simulink model "image_processing_system"  (Simulink 7.6)
settings: Solver=FixedStepDiscrete  StartTime=0.0  StopTime=inf  FixedStep=(1/19200)  RelTol=1e-3
undefined symbols (not defined in the file or in its folder): none, serial, videoinput
libraries: instrumentlib x2, vipsnks x1, imaqlib x1, vipstatistics x1
settings Model: Creator=jdoke  LastModifiedBy=Team10
settings DataIOCC: LimitDataPoints=off
settings OptimizationCC: InlineParams=on
settings DebuggingCC: SolverPrmCheckMsg=none  StrictBusMsg=Warning
settings ModelReferenceCC: ModelReferenceNumInstancesAllowed=Single

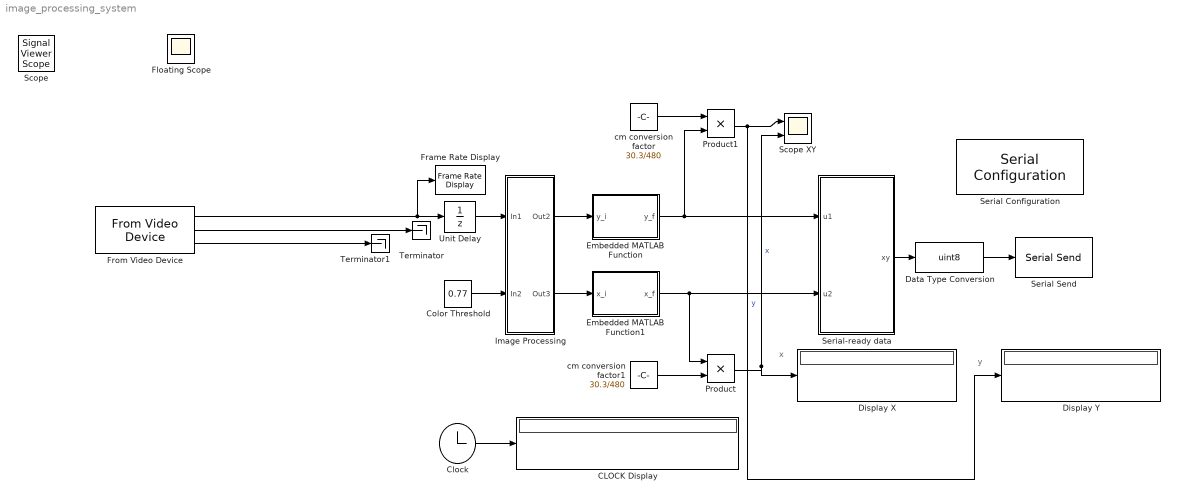
== system image_processing_system ==
  note: y
  note: x
  CLOCK Display : Display
  Clock : Clock
      settings: Decimation=10
  Color Threshold : Constant  Value=0.77
  Data Type Conversion : DataTypeConversion  OutDataTypeStr=uint8
  Display X : Display
  Display Y : Display
  Embedded MATLAB Function : Stateflow chart  TreatAsAtomicUnit=on
  Embedded MATLAB Function1 : Stateflow chart  TreatAsAtomicUnit=on
  Frame Rate Display : vipsnks/Frame Rate Display  DialogController=vipDDGCreate  DialogControllerArgs=DataTag0  UpdateRate=10
  From Video Device : imaqlib/From Video Device  DialogController=imaqcreatedialog  DialogControllerArgs=DataTag2  DeviceMenu=winvideo 1 (PC VGA Camer@ Plus)  Device=winvideo 1 (PC VGA Camer@ Plus)  ObjConstructor=videoinput('winvideo', 1)  VideoFormatMenu=RGB24_640x480  VideoFormat=RGB24_640x480  VideoSource=input1  ROIPosition=[0 0 480 480]  EnableHWTrigger=off  TriggerConfiguration=none/none  SampleTime=1/192  OutputPortsMode=Separate color signals  DataType=single  CanDoHWTrigger=no  ReturnedColorSpace=rgb  BlockHandle=31.001  ROIWidth=480  ROIHeight=480  ROIColumn=0  ROIRow=0  EngXMLPath=C:\Program Files\MATLAB\R2010b\toolbox\imaq\imaq\private  DevXMLPath=C:\Program Files\MATLAB\R2010b\toolbox\imaq\imaqadaptors\win32  EngLibPath=C:\Program Files\MATLAB\R2010b\toolbox\imaq\imaqblks\imaqmex\win32
  Image Processing : Subsystem
  Product : Product  RndMeth=Zero
  Product1 : Product  RndMeth=Zero
  Scope XY : Scope  NumInputPorts=2
      settings: TimeRange=10  YMin=8.3~6  YMax=9.45~15
  Serial Configuration : instrumentlib/Serial Configuration  Priority=-200000  DialogController=instrumentcreatedialog  DialogControllerArgs=DataTag4  ComPortMenu=COM1  ComPort=COM1  ObjConstructor=serial('COM1');  BaudRate=19200  DataBits=7  Parity=none  StopBits=1  FlowControl=none  Timeout=10  ByteOrder=LittleEndian
  Serial Send : instrumentlib/Serial Send  DialogController=instrumentcreatedialog  DialogControllerArgs=DataTag5  ComPortMenu=COM1  ComPort=COM1  ObjConstructor=serial('COM1');  Terminator=<none>  EnableBlockingMode=off
  Serial-ready data : Stateflow chart  TreatAsAtomicUnit=on
  Terminator : Terminator
  Terminator1 : Terminator
  Unit Delay : UnitDelay  SampleTime=1/192
  cm conversion factor : Constant  Value=30.3/480
  cm conversion factor1 : Constant  Value=30.3/480
  Floating Scope : Scope
      settings: Floating=on
  Scope : SignalViewerScope  IOType=viewer  RefreshTime=0.035000
      settings: TimeRange=10  YMin=-50  YMax=650
  wires:
  From Video Device/1 -> Frame Rate Display/1, Unit Delay/1
  Color Threshold/1 -> Image Processing/2(In2)
  Image Processing/1(Out2) -> Embedded MATLAB Function/1(y_i)
  Image Processing/2(Out3) -> Embedded MATLAB Function1/1(x_i)
  Serial-ready data/1(xy) -> Data Type Conversion/1
  Embedded MATLAB Function1/1(x_f) -> Product/1, Serial-ready data/2(u2)
  Embedded MATLAB Function/1(y_f) -> Product1/2, Serial-ready data/1(u1)
  Product1/1 -> Scope XY/1, Display Y/1  "y"
  Product/1 -> Scope XY/2, Display X/1  "x"
  cm conversion factor1/1 -> Product/2
  cm conversion factor/1 -> Product1/1
  From Video Device/2 -> Terminator/1
  From Video Device/3 -> Terminator1/1
  Clock/1 -> CLOCK Display/1
  Data Type Conversion/1 -> Serial Send/1
  Unit Delay/1 -> Image Processing/1(In1)

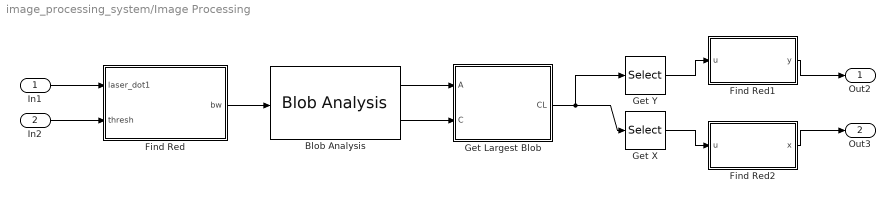
== system image_processing_system/Image Processing ==
  In1 : Inport
  In2 : Inport  Port=2
  Blob Analysis : vipstatistics/Blob Analysis  Tag=vipblks_row_conv  DialogController=vipDDGCreate  DialogControllerArgs=DataTag3  area=on  centroid=on  bBox=off  majorAxis=off  minorAxis=off  angle=off  eccentricity=off  equivDiameterSq=off  extent=off  perimeter=off  maxBlobs=10  warnIfNumBlobsExceeded=off  isCount=off  useMinArea=on  minArea=30  useMaxArea=off  maxArea=inf  excludeBorderBlob=off  outDT=double  isOutVarDim=off  isFill=on  fillValues=-10  conn=8  isLabel=off  outputMode=Binary point scaling  outputWordLength=32  outputFracLength=16  firstCoeffMode=Binary point scaling  firstCoeffWordLength=16  firstCoeffFracLength=14  secondCoeffMode=Binary point scaling  secondCoeffWordLength=32  secondCoeffFracLength=16  accumMode=Binary point scaling  accumWordLength=32  accumFracLength=0  prodOutputMode=Binary point scaling  prodOutputWordLength=32  prodOutputFracLength=16  roundingMode=Floor  overflowMode=off
  Find Red : Stateflow chart  TreatAsAtomicUnit=on
  Find Red1 : Stateflow chart  TreatAsAtomicUnit=on
  Find Red2 : Stateflow chart  TreatAsAtomicUnit=on
  Get Largest Blob : Stateflow chart  TreatAsAtomicUnit=on
  Get X : Selector  InputPortWidth=2  IndexOptions=Index vector (dialog)  Indices=[2]  OutputSizes=1
  Get Y : Selector  InputPortWidth=2  IndexOptions=Index vector (dialog)  Indices=[1]  OutputSizes=1
  Out2 : Outport
  Out3 : Outport  Port=2
  wires:
  Get Largest Blob/1(CL) -> Get X/1, Get Y/1
  In1/1 -> Find Red/1(laser_dot1)
  Get X/1 -> Find Red2/1(u)
  Get Y/1 -> Find Red1/1(u)
  Find Red1/1(y) -> Out2/1
  Find Red2/1(x) -> Out3/1
  In2/1 -> Find Red/2(thresh)
  Find Red/1(bw) -> Blob Analysis/1
  Blob Analysis/1 -> Get Largest Blob/1(A)
  Blob Analysis/2 -> Get Largest Blob/2(C)

== matlab function Image Processing/Get Largest Blob ==
  data: A input double; CL output double; C input double
function CL = getMax(A, C)
% getMax  Returns the centroid of the largest blob

%#eml

[~, id] = max(A);
CL = C(:, id);

== matlab function Image Processing/Find Red ==
  data: laser_dot1 input double; bw output double; thresh input double
function bw = findlaser(laser_dot1, thresh)
% This block supports the Embedded MATLAB subset.
% See the help menu for details. 

%% Extract each color
% Next we using indexing to extract three 2D matrices from the 3D image
% data corresponding to the red, green, and blue components of the image.
% r = laser_dot1(:,:,1);

%% Calculate Green
% Then we perform an arithmetic operation on the matrices as a whole to try
% to create one matrix that represents an intensity of green.

%justRed = r - g/8 -2*b/5;



%% Threshold the image
% Now we can set a threshold to separate the parts of the image that we
% consider to be red from the rest.
bw = laser_dot1 > thresh;

== matlab function Image Processing/Find Red1 ==
  data: u input double; y output double
function y = integ(u)

y = ceil(u);

end

== matlab function Image Processing/Find Red2 ==
  data: u input double; x output double
function x = integ(u)

x = ceil(u);

end

== matlab function Serial-ready data ==
  data: xy output double; u1 input double; u2 input double
function xy  = integ(u1,u2)

xy = [0,0,0,0,0,0,0,0];
y1 = 0; y2 = 0; y3 = 0; y4 = 0; 
x1 = 0; x2 = 0; x3 = 0; x4 = 0;

if u1 >=0 && u1 <= 127
    y1 = u1;
else
    y1 = 127;
    
    if u1 >= 127 && u1<= 255
        y2 = u1 - 127;
    else
        y2 = 127;
        
        if u1 >= 255 && u1<=383
            y3 = u1 - 254;
        else
            y3 = 127;
            
            if u1>=383 && u1<=480
                y4 = u1 - (383) + 2;
            end
        end
    end
end

% x - coordinate parsing

if u2 >=0 && u2 <= 127
    x1 = u2;
else
    x1 = 127;
    
    if u2 >= 127 && u2<= 255
        x2 = u2 - 127;
    else
        x2 = 127;
        
        if u2 >= 255 && u2<=383
            x3 = u2 - 254;
        else
            x3 = 127;
            
            if u2>=383 && u2<=480
                x4 = u2 - (383)+2;
            end
        end
    end
end

xy = [y1,y2,y3,y4,x1,x2,x3,x4];

end

== matlab function Embedded MATLAB Function ==
  data: y_i input double; y_f output double
function y_f = y_f(y_i)

 y_f = abs(y_i - 480);
 
end

== matlab function Embedded MATLAB Function1 ==
  data: x_i input double; x_f output double
function x_f = x_f(x_i)

 x_f = abs(x_i - 480);
 
end
